simulink model "bh_4bar_model_KIN"  (R2019a)
settings: Solver=ode45  StartTime=0.0  StopTime=20  MaxStep=0.1  RelTol=1e-3  EnableMultiTasking=on
values from neighbouring files (symbols this model uses):
  L1 = 0.4    [bh_4bar_kin_z_analysis_CLS.m]
  L2 = 1.4    [bh_4bar_kin_z_analysis_CLS.m]
  L3 = 1.2    [bh_4bar_kin_z_analysis_CLS.m]
  L4 = 1    [bh_4bar_kin_z_analysis_CLS.m]
  N = length(THE_DEG_ANG_VEC)    [bh_4bar_kin_z_analysis_CLS.m]
  X = my_stuff_T.theta_deg_vec    [bh_4bar_kin_z_analysis_CLS.m]
undefined symbols (not defined in the file or in its folder): H, joints, theta_0_rad, W, Y, Z
libraries: nesl_utility x27, sm_lib x17, simulink_extras x7, bh_4bar_SL_LIB x7, simulink x1
settings Model: EnablePacing=on  Creator=bhorton  LastModifiedBy=bhorton
settings DataIOCC: LimitDataPoints=on  ReturnWorkspaceOutputs=off
settings OptimizationCC: LifeSpan=inf
settings DebuggingCC: AllowSymbolicDim=off  PregeneratedLibrarySubsystemCodeDiagnostic=none  SFUnexpectedBacktrackingDiag=warning  SFNoUnconditionalDefaultTransitionDiag=warning  SFExecutionAtInitializationDiag=none  ArithmeticOperatorsInVariantConditions=warning
settings SFSimCC: SimUseLocalCustomCode=off
settings RTWCC: RTWUseLocalCustomCode=off
settings CodeAppCC: StateflowObjectComments=on
settings GRTTargetCC: TargetLangStandard=C89/C90 (ANSI)  GeneratePreprocessorConditionals=Disable all
settings ConfigComp: CovMetricSettings=dw  CovHtmlReporting=on  CovSaveCumulativeToWorkspaceVar=on  CovSaveSingleToWorkspaceVar=on  CovExternalEMLEnable=off  CovSFcnEnable=off
settings SimscapeCC: SimscapeNominalValues="[{\"value\":\"10\",\"unit\":\"V\"},{\"value\":\"1\",\"unit\":\"A\"},{\"value\":\"10\",\"unit\":\"N*m\"},{\"value\":\"10\",\"unit\":\"bar\"},{\"value\":\"100\",\"unit\":\"kJ/kg\"},{\"value\":\"1\",\"unit\":\"kW\"},{\"value\":\"300\",\"unit\":\"K\"},{\"value\":\"100\",\"unit\":\"cm^3/s\"},{\"value\":\"1\",\"unit\":\"kN\"},{\"value\":\"1\",\"unit\":\"g/cm^3\"},{\"value\":\"1\",\"unit\":\"l\"},{\"value\":\"1\",\"unit\":\"cm^2\"},{\"value\":\"60\",\"unit\":\"Hz\"}]"  SimscapeLogType=all  SimscapeLogDataHistory=10000
settings ConfigurationSet: Description=SimMechanics 2G
settings ExplorerConfigSet: InternalSimMechanicsExplorerSettings="<ExplorerConfiguration><canonicalview>default</canonicalview><AnimationSetting><BasePlaybackSpeed>1.0</BasePlaybackSpeed><PlaybackSpeedFactor>1.0</PlaybackSpeedFactor></AnimationSetting><TilePanel><TileInfo><Tiles Columns=\"1\" Count=\"1\" Rows=\"1\"><Column Weight=\"1\"/><Row Weight=\"1\"/><Tile Height=\"1\" Width=\"1\" X=\"0\" Y=\"0\"/></Tiles></TileInfo><SceneInfo><SceneViewer><BGColor><R>0.60000002384185791</R><G>0.60000002384185791</G><B>0.60000002384185791</B></BGColor><Camera><DoPerspective>off</DoPerspective><Position><X>0.027900076379062555</X><Y>-0.43953442521543673</Y><Z>1.15928585903234671</Z></Position><Center><X>0.027900076379062555</X><Y>-0.43953442521543673</Y><Z>-0.00499998996240980098</Z></Center><Up><X>0</X><Y>1</Y><Z>-0</Z></Up><ViewLimDist>1</ViewLimDist><YLim>2.16648122412032906</YLim><XLim>2.57652145580412029</XLim></Camera></SceneViewer></SceneInfo></TilePanel><MechEditorPanel><Cameras/><GfxPanelCameraMap/><VideoCreator><PlaybackSpeedRatio>1.0</PlaybackSpeedRatio><FrameRate>30</FrameRate><VideoFormat>Motion JPEG AVI</VideoFormat><FrameSize>auto</FrameSize></VideoCreator></MechEditorPanel></ExplorerConfiguration>"

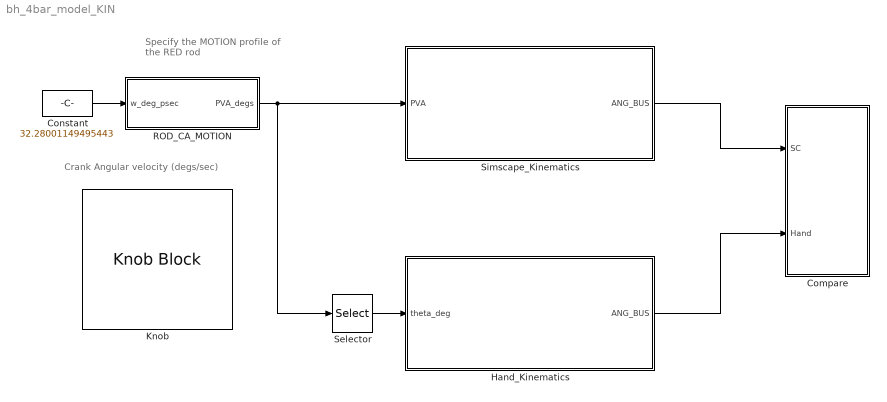
== system bh_4bar_model_KIN ==
  note: Crank Angular velocity (degs/sec)
  note: Specify the MOTION
      | profile of the RED rod
  Compare : Subsystem
  Constant : Constant  Value=32.28001149495443
  Hand_Kinematics : Subsystem
  Knob : KnobBlock
  ROD_CA_MOTION : Subsystem
  Selector : Selector  InputPortWidth=3  IndexOptions=Index vector (dialog)  Indices=1  OutputSizes=1
  Simscape_Kinematics : Subsystem
  wires:
  ROD_CA_MOTION/1(PVA_degs) -> Simscape_Kinematics/1(PVA), Selector/1
  Selector/1 -> Hand_Kinematics/1(theta_deg)
  Simscape_Kinematics/1(ANG_BUS) -> Compare/1(SC)
  Hand_Kinematics/1(ANG_BUS) -> Compare/2(Hand)
  Constant/1 -> ROD_CA_MOTION/1(w_deg_psec)

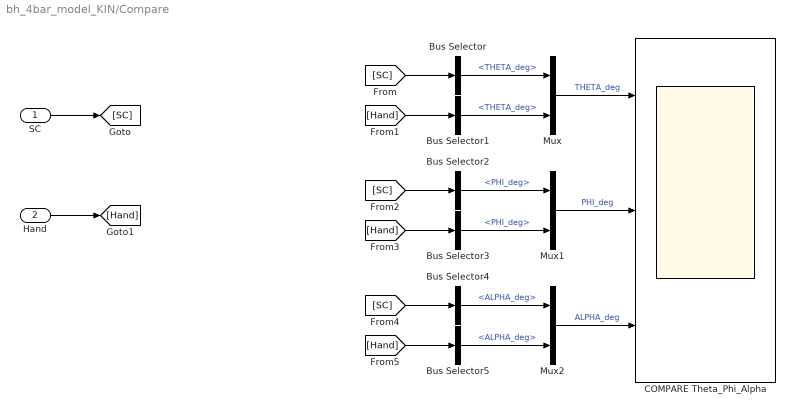
== system bh_4bar_model_KIN/Compare ==
  SC : Inport
  Hand : Inport  Port=2
  Bus Selector : BusSelector  OutputSignals=THETA_deg
  Bus Selector1 : BusSelector  OutputSignals=THETA_deg
  Bus Selector2 : BusSelector  OutputSignals=PHI_deg
  Bus Selector3 : BusSelector  OutputSignals=PHI_deg
  Bus Selector4 : BusSelector  OutputSignals=ALPHA_deg
  Bus Selector5 : BusSelector  OutputSignals=ALPHA_deg
  COMPARE Theta_Phi_Alpha : Scope  NumInputPorts=3
  Mux : Mux  Inputs=2
  Mux1 : Mux  Inputs=2
  Mux2 : Mux  Inputs=2
  wires:
  Hand/1 -> [Hand]
  SC/1 -> [SC]
  Mux/1 -> COMPARE Theta_Phi_Alpha/1  "THETA_deg"
  [SC] -> Bus Selector/1
  Bus Selector/1 -> Mux/1  "<THETA_deg>"
  [Hand] -> Bus Selector1/1
  Bus Selector1/1 -> Mux/2  "<THETA_deg>"
  Mux1/1 -> COMPARE Theta_Phi_Alpha/2  "PHI_deg"
  [SC] -> Bus Selector2/1
  Bus Selector3/1 -> Mux1/2  "<PHI_deg>"
  [Hand] -> Bus Selector3/1
  Bus Selector2/1 -> Mux1/1  "<PHI_deg>"
  Mux2/1 -> COMPARE Theta_Phi_Alpha/3  "ALPHA_deg"
  [Hand] -> Bus Selector5/1
  [SC] -> Bus Selector4/1
  Bus Selector5/1 -> Mux2/2  "<ALPHA_deg>"
  Bus Selector4/1 -> Mux2/1  "<ALPHA_deg>"

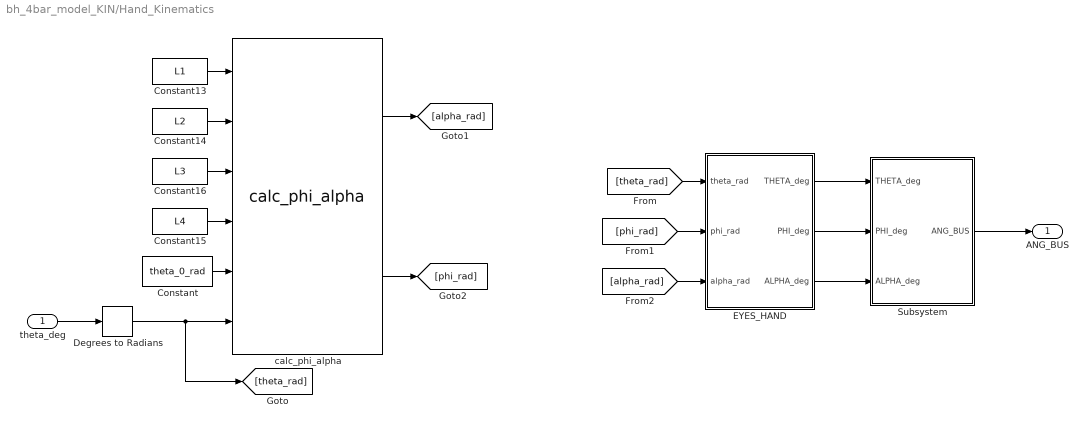
== system bh_4bar_model_KIN/Hand_Kinematics ==
  theta_deg : Inport
  Constant : Constant  Value=theta_0_rad
  Constant13 : Constant  Value=L1
  Constant14 : Constant  Value=L2
  Constant15 : Constant  Value=L4
  Constant16 : Constant  Value=L3
  Degrees to Radians : simulink_extras/Transformations/Degrees to Radians
  EYES_HAND : Subsystem
  Subsystem : Subsystem
  calc_phi_alpha : bh_4bar_SL_LIB/4bar_basics/calc_phi_alpha  SystemSampleTime=-1
  ANG_BUS : Outport
  wires:
  Constant14/1 -> calc_phi_alpha/2
  Constant13/1 -> calc_phi_alpha/1
  Constant15/1 -> calc_phi_alpha/4
  Constant16/1 -> calc_phi_alpha/3
  Degrees to Radians/1 -> [theta_rad], calc_phi_alpha/6
  theta_deg/1 -> Degrees to Radians/1
  EYES_HAND/1(THETA_deg) -> Subsystem/1(THETA_deg)
  EYES_HAND/3(ALPHA_deg) -> Subsystem/3(ALPHA_deg)
  EYES_HAND/2(PHI_deg) -> Subsystem/2(PHI_deg)
  [phi_rad] -> EYES_HAND/2(phi_rad)
  Subsystem/1(ANG_BUS) -> ANG_BUS/1
  [alpha_rad] -> EYES_HAND/3(alpha_rad)
  [theta_rad] -> EYES_HAND/1(theta_rad)
  calc_phi_alpha/2 -> [phi_rad]
  calc_phi_alpha/1 -> [alpha_rad]
  Constant/1 -> calc_phi_alpha/5

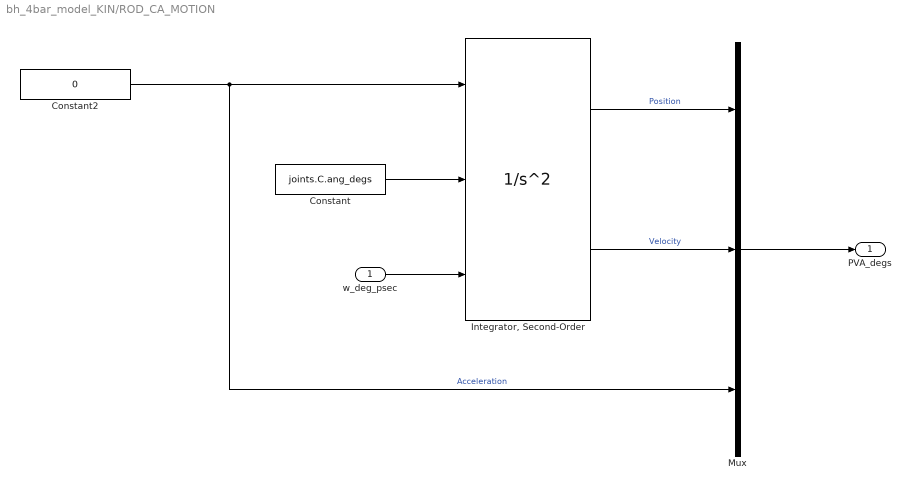
== system bh_4bar_model_KIN/ROD_CA_MOTION ==
  w_deg_psec : Inport
  Constant : Constant  Value=joints.C.ang_degs
  Constant2 : Constant  Value=0
  "Integrator, Second-Order" : SecondOrderIntegrator  ICSourceX=external  ICSourceDXDT=external
  Mux : Mux  Inputs=3
  PVA_degs : Outport
  wires:
  Constant2/1 -> Mux/3, "Integrator, Second-Order"/1  "Acceleration"
  w_deg_psec/1 -> "Integrator, Second-Order"/3
  Constant/1 -> "Integrator, Second-Order"/2
  "Integrator, Second-Order"/1 -> Mux/1  "Position"
  "Integrator, Second-Order"/2 -> Mux/2  "Velocity"
  Mux/1 -> PVA_degs/1

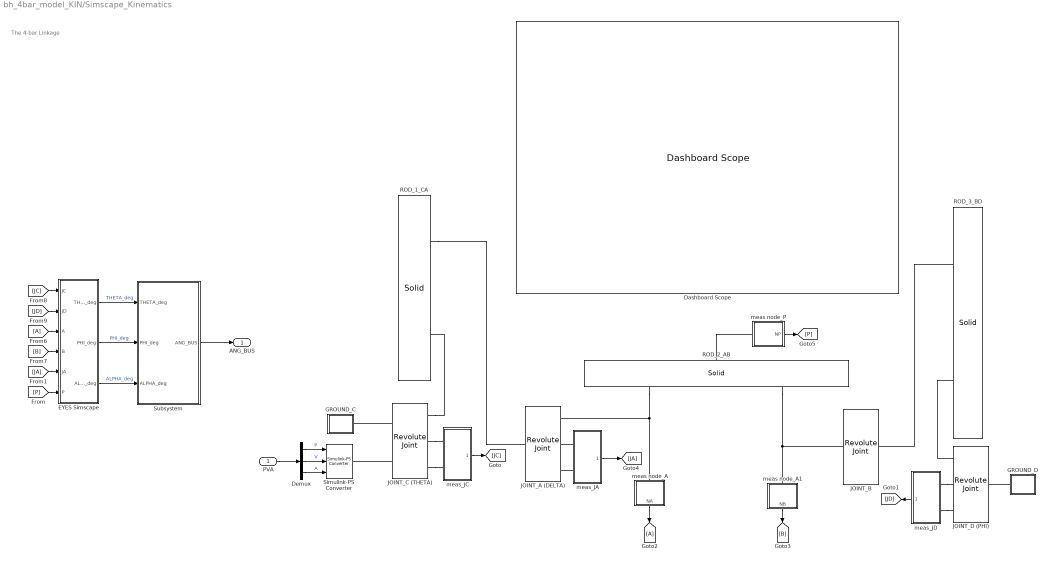
== system bh_4bar_model_KIN/Simscape_Kinematics ==
  note: The 4-bar Linkage
  PVA : Inport
  Dashboard Scope : DashboardScope
  Demux : Demux  Outputs=3
  EYES Simscape : Subsystem
  GROUND_C : Subsystem
  GROUND_D : Subsystem
  JOINT_A (DELTA) : sm_lib/Joints/Revolute Joint  SenseConstraintForce=off  SenseConstraintForceX=off  SenseConstraintForceY=off  SenseConstraintForceZ=off  SenseConstraintTorque=off  SenseConstraintTorqueX=off  SenseConstraintTorqueY=off  SenseConstraintTorqueZ=off  SenseTotalForce=off  SenseTotalForceX=off  SenseTotalForceY=off  SenseTotalForceZ=off  SenseTotalTorque=off  SenseTotalTorqueX=off  SenseTotalTorqueY=off  SenseTotalTorqueZ=off  CompositeWrenchDir=FollowerOnBase  CompositeWrenchFrame=BaseFrame  EquilibriumPosition=0  EquilibriumPositionUnits=deg  SpringStiffness=0  SpringStiffnessUnits=N*m/deg  DampingCoefficient=0  DampingCoefficientUnits=N*m/(deg/s)  TorqueActuationMode=NoTorque  MotionActuationMode=ComputedMotion  SensePosition=on  SenseVelocity=on  SenseAcceleration=off  SenseTorqueForce=off  SenseLowerLimitTorqueForce=off  SenseUpperLimitTorqueForce=off  LowerLimitSpecify=off  LowerLimitBound=-90  LowerLimitBoundUnits=deg  LowerLimitStiffness=1e4  LowerLimitStiffnessUnits=N*m/deg  LowerLimitDamping=10  LowerLimitDampingUnits=N*m/(deg/s)  LowerLimitTransitionRegionWidth=0.1  LowerLimitTransitionRegionWidthUnits=deg  UpperLimitSpecify=off  UpperLimitBound=90  UpperLimitBoundUnits=deg  UpperLimitStiffness=1e4  UpperLimitStiffnessUnits=N*m/deg  UpperLimitDamping=10  UpperLimitDampingUnits=N*m/(deg/s)  UpperLimitTransitionRegionWidth=0.1  UpperLimitTransitionRegionWidthUnits=deg  PositionTargetSpecify=off  PositionTargetPriority=High  PositionTargetValue=0  PositionTargetValueUnits=deg  VelocityTargetSpecify=off  VelocityTargetPriority=High  VelocityTargetValue=0  VelocityTargetValueUnits=deg/s
  JOINT_B : sm_lib/Joints/Revolute Joint  SenseConstraintForce=off  SenseConstraintForceX=off  SenseConstraintForceY=off  SenseConstraintForceZ=off  SenseConstraintTorque=off  SenseConstraintTorqueX=off  SenseConstraintTorqueY=off  SenseConstraintTorqueZ=off  SenseTotalForce=off  SenseTotalForceX=off  SenseTotalForceY=off  SenseTotalForceZ=off  SenseTotalTorque=off  SenseTotalTorqueX=off  SenseTotalTorqueY=off  SenseTotalTorqueZ=off  CompositeWrenchDir=FollowerOnBase  CompositeWrenchFrame=BaseFrame  EquilibriumPosition=0  EquilibriumPositionUnits=deg  SpringStiffness=0  SpringStiffnessUnits=N*m/deg  DampingCoefficient=0  DampingCoefficientUnits=N*m/(deg/s)  TorqueActuationMode=NoTorque  MotionActuationMode=ComputedMotion  SensePosition=off  SenseVelocity=off  SenseAcceleration=off  SenseTorqueForce=off  SenseLowerLimitTorqueForce=off  SenseUpperLimitTorqueForce=off  LowerLimitSpecify=off  LowerLimitBound=-90  LowerLimitBoundUnits=deg  LowerLimitStiffness=1e4  LowerLimitStiffnessUnits=N*m/deg  LowerLimitDamping=10  LowerLimitDampingUnits=N*m/(deg/s)  LowerLimitTransitionRegionWidth=0.1  LowerLimitTransitionRegionWidthUnits=deg  UpperLimitSpecify=off  UpperLimitBound=90  UpperLimitBoundUnits=deg  UpperLimitStiffness=1e4  UpperLimitStiffnessUnits=N*m/deg  UpperLimitDamping=10  UpperLimitDampingUnits=N*m/(deg/s)  UpperLimitTransitionRegionWidth=0.1  UpperLimitTransitionRegionWidthUnits=deg  PositionTargetSpecify=off  PositionTargetPriority=High  PositionTargetValue=0  PositionTargetValueUnits=deg  VelocityTargetSpecify=off  VelocityTargetPriority=High  VelocityTargetValue=0  VelocityTargetValueUnits=deg/s
  JOINT_C (THETA) : sm_lib/Joints/Revolute Joint  SenseConstraintForce=off  SenseConstraintForceX=off  SenseConstraintForceY=off  SenseConstraintForceZ=off  SenseConstraintTorque=off  SenseConstraintTorqueX=off  SenseConstraintTorqueY=off  SenseConstraintTorqueZ=off  SenseTotalForce=off  SenseTotalForceX=off  SenseTotalForceY=off  SenseTotalForceZ=off  SenseTotalTorque=off  SenseTotalTorqueX=off  SenseTotalTorqueY=off  SenseTotalTorqueZ=off  CompositeWrenchDir=FollowerOnBase  CompositeWrenchFrame=BaseFrame  EquilibriumPosition=0  EquilibriumPositionUnits=deg  SpringStiffness=0  SpringStiffnessUnits=N*m/deg  DampingCoefficient=0  DampingCoefficientUnits=N*m/(deg/s)  TorqueActuationMode=ComputedTorque  MotionActuationMode=InputMotion  SensePosition=on  SenseVelocity=on  SenseAcceleration=off  SenseTorqueForce=off  SenseLowerLimitTorqueForce=off  SenseUpperLimitTorqueForce=off  LowerLimitSpecify=off  LowerLimitBound=-90  LowerLimitBoundUnits=deg  LowerLimitStiffness=1e4  LowerLimitStiffnessUnits=N*m/deg  LowerLimitDamping=10  LowerLimitDampingUnits=N*m/(deg/s)  LowerLimitTransitionRegionWidth=0.1  LowerLimitTransitionRegionWidthUnits=deg  UpperLimitSpecify=off  UpperLimitBound=90  UpperLimitBoundUnits=deg  UpperLimitStiffness=1e4  UpperLimitStiffnessUnits=N*m/deg  UpperLimitDamping=10  UpperLimitDampingUnits=N*m/(deg/s)  UpperLimitTransitionRegionWidth=0.1  UpperLimitTransitionRegionWidthUnits=deg  PositionTargetSpecify=on  PositionTargetPriority=High  PositionTargetValue=joints.C.ang_degs  PositionTargetValueUnits=deg  VelocityTargetSpecify=on  VelocityTargetPriority=High  VelocityTargetValue=joints.C.vel_degs  VelocityTargetValueUnits=deg/s
      settings: AttributesFormatString=|
      | init_pos =%<PositionTargetValue>
      | %<PositionTargetValueUnits>
  JOINT_D (PHI) : sm_lib/Joints/Revolute Joint  SenseConstraintForce=off  SenseConstraintForceX=off  SenseConstraintForceY=off  SenseConstraintForceZ=off  SenseConstraintTorque=off  SenseConstraintTorqueX=off  SenseConstraintTorqueY=off  SenseConstraintTorqueZ=off  SenseTotalForce=off  SenseTotalForceX=off  SenseTotalForceY=off  SenseTotalForceZ=off  SenseTotalTorque=off  SenseTotalTorqueX=off  SenseTotalTorqueY=off  SenseTotalTorqueZ=off  CompositeWrenchDir=FollowerOnBase  CompositeWrenchFrame=BaseFrame  EquilibriumPosition=0  EquilibriumPositionUnits=deg  SpringStiffness=0  SpringStiffnessUnits=N*m/deg  DampingCoefficient=0  DampingCoefficientUnits=N*m/(deg/s)  TorqueActuationMode=NoTorque  MotionActuationMode=ComputedMotion  SensePosition=on  SenseVelocity=on  SenseAcceleration=off  SenseTorqueForce=off  SenseLowerLimitTorqueForce=off  SenseUpperLimitTorqueForce=off  LowerLimitSpecify=off  LowerLimitBound=-90  LowerLimitBoundUnits=deg  LowerLimitStiffness=1e4  LowerLimitStiffnessUnits=N*m/deg  LowerLimitDamping=10  LowerLimitDampingUnits=N*m/(deg/s)  LowerLimitTransitionRegionWidth=0.1  LowerLimitTransitionRegionWidthUnits=deg  UpperLimitSpecify=off  UpperLimitBound=90  UpperLimitBoundUnits=deg  UpperLimitStiffness=1e4  UpperLimitStiffnessUnits=N*m/deg  UpperLimitDamping=10  UpperLimitDampingUnits=N*m/(deg/s)  UpperLimitTransitionRegionWidth=0.1  UpperLimitTransitionRegionWidthUnits=deg  PositionTargetSpecify=on  PositionTargetPriority=High  PositionTargetValue=joints.D.ang_degs  PositionTargetValueUnits=deg  VelocityTargetSpecify=off  VelocityTargetPriority=High  VelocityTargetValue=0  VelocityTargetValueUnits=deg/s
      settings: AttributesFormatString=|
      | init_pos =%<PositionTargetValue>
      | %<PositionTargetValueUnits>
  ROD_1_CA : sm_lib/Body Elements/Solid  InertiaType=CalculateFromGeometry  Mass=1  MassUnits=kg  CenterOfMass=[0 0 0]  CenterOfMassUnits=m  MomentsOfInertia=[1 1 1]  MomentsOfInertiaUnits=kg*m^2  ProductsOfInertia=[0 0 0]  ProductsOfInertiaUnits=kg*m^2  BasedOnType=Density  Density=density  DensityUnits=kg/m^3  DoExposeReferenceFrame=on  SerializedFrames=<Frames><Frame><Id>Frame2</Id><Value><Name>A</Name><Origin><Source>GeometricFeature</Source><FeatureName>+z +x curve</FeatureName></Origin><PrimaryAxis><DefinedDirection>+Z</DefinedDirection><Source>ReferenceFrame</Source><SourceDirection>+Z</SourceDirection><FeatureName></FeatureName></PrimaryAxis><SecondaryAxis><DefinedDirection>+X</DefinedDirection><Source>ReferenceFrame</Source><SourceDirection>+X</SourceDirection><FeatureName></FeatureName></SecondaryAxis></Value></Frame><Frame><Id>Frame3</Id><Value><Name>C</Name><Origin><Source>GeometricFeature</Source><FeatureName>+z -x curve</FeatureName></Origin><PrimaryAxis><DefinedDirection>+Z</DefinedDirection><Source>ReferenceFrame</Source><SourceDirection>+Z</SourceDirection><FeatureName></FeatureName></PrimaryAxis><SecondaryAxis><DefinedDirection>+X</DefinedDirection><Source>ReferenceFrame</Source><SourceDirection>+X</SourceDirection><FeatureName></FeatureName></SecondaryAxis></Value></Frame></Frames>  GraphicType=FromGeometry  MarkerShape=Sphere  MarkerSize=10  GraphicVisPropType=SimpleVisualProperties  GraphicDiffuseColor=[1.0 0.4 0.6]  GraphicSpecularColor=[0.5 0.5 0.5 1.0]  GraphicAmbientColor=[0.15 0.15 0.15 1.0]  GraphicEmissiveColor=[0.0 0.0 0.0 1.0]  GraphicShininess=75  GraphicOpacity=1.0  GeometryShape=Brick  RectangleSize=[1 1]  RectangleSizeUnits=m  BrickDimensions=[L1,H,W]  BrickDimensionUnits=m  CylinderRadius=1  CylinderRadiusUnits=m  CylinderLength=1  CylinderLengthUnits=m  SphereRadius=1  SphereRadiusUnits=m  EllipsoidRadii=[1 1 1]  EllipsoidRadiiUnits=m  ExtrusionCrossSection=[1 1; -1 1; -1 -1; 1 -1]  ExtrusionCrossSectionUnits=m  ExtrusionLength=1  ExtrusionLengthUnits=m  PolygonNumSides=3  PolygonOuterRadius=1  PolygonOuterRadiusUnits=m  ExtGeomFileType=STEP  ExtGeomFileUnits=m  RevolutionCrossSection=[1 1; 1 -1; 2 -1; 2 1]  RevolutionCrossSectionUnits=m  RevolutionExtent=Full  RevolutionAngle=180  RevolutionAngleUnits=deg
  ROD_2_AB : sm_lib/Body Elements/Solid  InertiaType=CalculateFromGeometry  Mass=1  MassUnits=kg  CenterOfMass=[0 0 0]  CenterOfMassUnits=m  MomentsOfInertia=[1 1 1]  MomentsOfInertiaUnits=kg*m^2  ProductsOfInertia=[0 0 0]  ProductsOfInertiaUnits=kg*m^2  BasedOnType=Density  Density=density  DensityUnits=kg/m^3  DoExposeReferenceFrame=on  SerializedFrames=<Frames><Frame><Id>Frame1</Id><Value><Name>A</Name><Origin><Source>GeometricFeature</Source><FeatureName>+z -x curve</FeatureName></Origin><PrimaryAxis><DefinedDirection>+Z</DefinedDirection><Source>ReferenceFrame</Source><SourceDirection>+Z</SourceDirection><FeatureName></FeatureName></PrimaryAxis><SecondaryAxis><DefinedDirection>+X</DefinedDirection><Source>ReferenceFrame</Source><SourceDirection>+X</SourceDirection><FeatureName></FeatureName></SecondaryAxis></Value></Frame><Frame><Id>Frame2</Id><Value><Name>B</Name><Origin><Source>GeometricFeature</Source><FeatureName>+z +x curve</FeatureName></Origin><PrimaryAxis><DefinedDirection>+Z</DefinedDirection><Source>ReferenceFrame</Source><SourceDirection>+Z</SourceDirection><FeatureName></FeatureName></PrimaryAxis><SecondaryAxis><DefinedDirection>+X</DefinedDirection><Source>ReferenceFrame</Source><SourceDirection>+X</SourceDirection><FeatureName></FeatureName></SecondaryAxis></Value></Frame></Frames>  GraphicType=FromGeometry  MarkerShape=Sphere  MarkerSize=10  GraphicVisPropType=SimpleVisualProperties  GraphicDiffuseColor=[0.0 1.0 0.2]  GraphicSpecularColor=[0.5 0.5 0.5 1.0]  GraphicAmbientColor=[0.15 0.15 0.15 1.0]  GraphicEmissiveColor=[0.0 0.0 0.0 1.0]  GraphicShininess=75  GraphicOpacity=1.0  GeometryShape=Brick  RectangleSize=[1 1]  RectangleSizeUnits=m  BrickDimensions=[L2,H,W]  BrickDimensionUnits=m  CylinderRadius=1  CylinderRadiusUnits=m  CylinderLength=1  CylinderLengthUnits=m  SphereRadius=1  SphereRadiusUnits=m  EllipsoidRadii=[1 1 1]  EllipsoidRadiiUnits=m  ExtrusionCrossSection=[1 1; -1 1; -1 -1; 1 -1]  ExtrusionCrossSectionUnits=m  ExtrusionLength=1  ExtrusionLengthUnits=m  PolygonNumSides=3  PolygonOuterRadius=1  PolygonOuterRadiusUnits=m  ExtGeomFileType=STEP  ExtGeomFileUnits=m  RevolutionCrossSection=[1 1; 1 -1; 2 -1; 2 1]  RevolutionCrossSectionUnits=m  RevolutionExtent=Full  RevolutionAngle=180  RevolutionAngleUnits=deg
  ROD_3_BD : sm_lib/Body Elements/Solid  InertiaType=CalculateFromGeometry  Mass=1  MassUnits=kg  CenterOfMass=[0 0 0]  CenterOfMassUnits=m  MomentsOfInertia=[1 1 1]  MomentsOfInertiaUnits=kg*m^2  ProductsOfInertia=[0 0 0]  ProductsOfInertiaUnits=kg*m^2  BasedOnType=Density  Density=density  DensityUnits=kg/m^3  DoExposeReferenceFrame=on  SerializedFrames=<Frames><Frame><Id>Frame1</Id><Value><Name>B</Name><Origin><Source>GeometricFeature</Source><FeatureName>+z +x curve</FeatureName></Origin><PrimaryAxis><DefinedDirection>+Z</DefinedDirection><Source>ReferenceFrame</Source><SourceDirection>+Z</SourceDirection><FeatureName></FeatureName></PrimaryAxis><SecondaryAxis><DefinedDirection>+X</DefinedDirection><Source>ReferenceFrame</Source><SourceDirection>+X</SourceDirection><FeatureName></FeatureName></SecondaryAxis></Value></Frame><Frame><Id>Frame2</Id><Value><Name>D</Name><Origin><Source>GeometricFeature</Source><FeatureName>+z -x curve</FeatureName></Origin><PrimaryAxis><DefinedDirection>+Z</DefinedDirection><Source>ReferenceFrame</Source><SourceDirection>+Z</SourceDirection><FeatureName></FeatureName></PrimaryAxis><SecondaryAxis><DefinedDirection>+X</DefinedDirection><Source>ReferenceFrame</Source><SourceDirection>+X</SourceDirection><FeatureName></FeatureName></SecondaryAxis></Value></Frame></Frames>  GraphicType=FromGeometry  MarkerShape=Sphere  MarkerSize=10  GraphicVisPropType=SimpleVisualProperties  GraphicDiffuseColor=[0.2 0.2 1.0]  GraphicSpecularColor=[0.5 0.5 0.5 1.0]  GraphicAmbientColor=[0.15 0.15 0.15 1.0]  GraphicEmissiveColor=[0.0 0.0 0.0 1.0]  GraphicShininess=75  GraphicOpacity=1.0  GeometryShape=Brick  RectangleSize=[1 1]  RectangleSizeUnits=m  BrickDimensions=[L3,H,W]  BrickDimensionUnits=m  CylinderRadius=1  CylinderRadiusUnits=m  CylinderLength=1  CylinderLengthUnits=m  SphereRadius=1  SphereRadiusUnits=m  EllipsoidRadii=[1 1 1]  EllipsoidRadiiUnits=m  ExtrusionCrossSection=[1 1; -1 1; -1 -1; 1 -1]  ExtrusionCrossSectionUnits=m  ExtrusionLength=1  ExtrusionLengthUnits=m  PolygonNumSides=3  PolygonOuterRadius=1  PolygonOuterRadiusUnits=m  ExtGeomFileType=STEP  ExtGeomFileUnits=m  RevolutionCrossSection=[1 1; 1 -1; 2 -1; 2 1]  RevolutionCrossSectionUnits=m  RevolutionExtent=Full  RevolutionAngle=180  RevolutionAngleUnits=deg
  Simulink-PS Converter : nesl_utility/Simulink-PS Converter  PhysicalDomain=network_engine_domain  SubClassName=ps_input  LeftPortType=input  RightPortType=output  PseudoPeriodic=off  Frequencies=[]  NoiseDistribution=none  NoiseParameters=[]  Unit=deg  AffineConversion=off  FilteringAndDerivatives=provide  SimscapeFilterOrder=1  InputFilterTimeConstant=0.001  UdotUserProvided=2
  Subsystem : Subsystem
  meas node_A : Subsystem
  meas node_A1 : Subsystem
  meas node_P : Subsystem
  meas_JA : Subsystem
  meas_JC : Subsystem
  meas_JD : Subsystem
  ANG_BUS : Outport
  wires:
  EYES Simscape/1(THETA_deg) -> Subsystem/1(THETA_deg)  "THETA_deg"
  Demux/2 -> Simulink-PS Converter/2  "V"
  Demux/1 -> Simulink-PS Converter/1  "P"
  meas_JD/1(PV_BUS) -> [JD]
  meas node_A/1(NA) -> [A]
  Subsystem/1(ANG_BUS) -> ANG_BUS/1
  [A] -> EYES Simscape/3(A)
  meas node_A1/1(NB) -> [B]
  [JA] -> EYES Simscape/5(JA)
  PVA/1 -> Demux/1
  meas_JC/1(PV_BUS) -> [JC]
  [JD] -> EYES Simscape/2(JD)
  Demux/3 -> Simulink-PS Converter/3  "A"
  EYES Simscape/2(PHI_deg) -> Subsystem/2(PHI_deg)  "PHI_deg"
  meas_JA/1(PV_BUS) -> [JA]
  [JC] -> EYES Simscape/1(JC)
  [B] -> EYES Simscape/4(B)
  EYES Simscape/3(ALPHA_deg) -> Subsystem/3(ALPHA_deg)  "ALPHA_deg"
  meas node_P/1(NP) -> [P]
  [P] -> EYES Simscape/6(P)
  connections:
  meas node_A/LConn1 -- ROD_2_AB/LConn1 -- JOINT_A (DELTA)/RConn1
  ROD_3_BD/LConn1 -- JOINT_B/RConn1
  JOINT_C (THETA)/LConn2 -- Simulink-PS Converter/RConn1
  JOINT_D (PHI)/RConn1 -- ROD_3_BD/LConn2
  ROD_2_AB/LConn2 -- meas node_A1/LConn1 -- JOINT_B/LConn1
  GROUND_D/RConn1 -- JOINT_D (PHI)/LConn1
  JOINT_C (THETA)/LConn1 -- GROUND_C/RConn1
  meas_JA/LConn1 -- JOINT_A (DELTA)/RConn2
  JOINT_C (THETA)/RConn3 -- meas_JC/LConn2
  meas_JD/LConn2 -- JOINT_D (PHI)/RConn3
  JOINT_C (THETA)/RConn2 -- meas_JC/LConn1
  meas_JD/LConn1 -- JOINT_D (PHI)/RConn2
  meas_JA/LConn2 -- JOINT_A (DELTA)/RConn3
  ROD_1_CA/LConn1 -- JOINT_A (DELTA)/LConn1
  JOINT_C (THETA)/RConn1 -- ROD_1_CA/LConn2
  ROD_2_AB/RConn1 -- meas node_P/LConn1

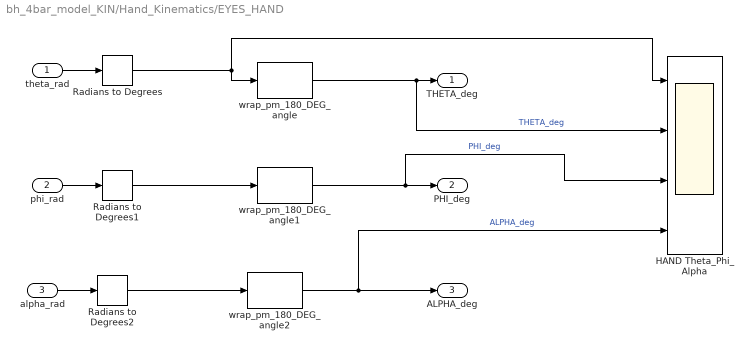
== system bh_4bar_model_KIN/Hand_Kinematics/EYES_HAND ==
  theta_rad : Inport
  phi_rad : Inport  Port=2
  alpha_rad : Inport  Port=3
  HAND Theta_Phi_Alpha : Scope  NumInputPorts=4
  Radians to Degrees : simulink_extras/Transformations/Radians to Degrees
  Radians to Degrees1 : simulink_extras/Transformations/Radians to Degrees
  Radians to Degrees2 : simulink_extras/Transformations/Radians to Degrees
  wrap_pm_180_DEG_angle : bh_4bar_SL_LIB/4bar_basics/wrap_pm_180_DEG_angle  SystemSampleTime=-1
  wrap_pm_180_DEG_angle1 : bh_4bar_SL_LIB/4bar_basics/wrap_pm_180_DEG_angle  SystemSampleTime=-1
  wrap_pm_180_DEG_angle2 : bh_4bar_SL_LIB/4bar_basics/wrap_pm_180_DEG_angle  SystemSampleTime=-1
  THETA_deg : Outport
  PHI_deg : Outport  Port=2
  ALPHA_deg : Outport  Port=3
  wires:
  theta_rad/1 -> Radians to Degrees/1
  alpha_rad/1 -> Radians to Degrees2/1
  phi_rad/1 -> Radians to Degrees1/1
  Radians to Degrees/1 -> wrap_pm_180_DEG_angle/1, HAND Theta_Phi_Alpha/1
  Radians to Degrees1/1 -> wrap_pm_180_DEG_angle1/1
  Radians to Degrees2/1 -> wrap_pm_180_DEG_angle2/1
  wrap_pm_180_DEG_angle/1 -> HAND Theta_Phi_Alpha/2, THETA_deg/1  "THETA_deg"
  wrap_pm_180_DEG_angle1/1 -> HAND Theta_Phi_Alpha/3, PHI_deg/1  "PHI_deg"
  wrap_pm_180_DEG_angle2/1 -> HAND Theta_Phi_Alpha/4, ALPHA_deg/1  "ALPHA_deg"

== system bh_4bar_model_KIN/Hand_Kinematics/Subsystem ==
  THETA_deg : Inport
  PHI_deg : Inport  Port=2
  ALPHA_deg : Inport  Port=3
  Bus Creator : BusCreator  Inputs=3
  ANG_BUS : Outport
  wires:
  ALPHA_deg/1 -> Bus Creator/3  "ALPHA_deg"
  PHI_deg/1 -> Bus Creator/2  "PHI_deg"
  THETA_deg/1 -> Bus Creator/1  "THETA_deg"
  Bus Creator/1 -> ANG_BUS/1

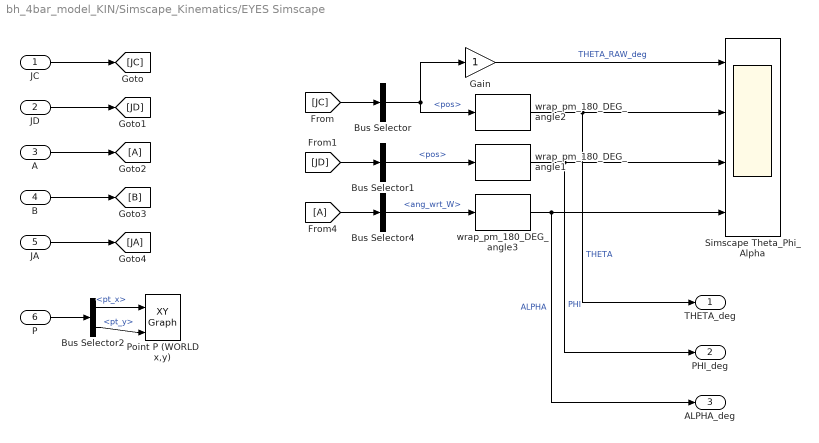
== system bh_4bar_model_KIN/Simscape_Kinematics/EYES Simscape ==
  JC : Inport
  JD : Inport  Port=2
  A : Inport  Port=3
  B : Inport  Port=4
  JA : Inport  Port=5
  P : Inport  Port=6
  Bus Selector : BusSelector  OutputSignals=pos
  Bus Selector1 : BusSelector  OutputSignals=pos
  Bus Selector2 : BusSelector  OutputSignals=pt_x,pt_y
  Bus Selector4 : BusSelector  OutputSignals=ang_wrt_W
  Gain : Gain
  Point P (WORLD x,y) : simulink/Sinks/XY Graph  xmin=-1*(L1+0.5*L2)  xmax=(L1+0.5*L2)  ymin=-1*max([L1, L3])  ymax=max([L1, L3])  st=-1
  Simscape Theta_Phi_Alpha : Scope  NumInputPorts=4
  wrap_pm_180_DEG_angle1 : bh_4bar_SL_LIB/4bar_basics/wrap_pm_180_DEG_angle  SystemSampleTime=-1
  wrap_pm_180_DEG_angle2 : bh_4bar_SL_LIB/4bar_basics/wrap_pm_180_DEG_angle  SystemSampleTime=-1
  wrap_pm_180_DEG_angle3 : bh_4bar_SL_LIB/4bar_basics/wrap_pm_180_DEG_angle  SystemSampleTime=-1
  THETA_deg : Outport
  PHI_deg : Outport  Port=2
  ALPHA_deg : Outport  Port=3
  wires:
  B/1 -> [B]
  A/1 -> [A]
  JD/1 -> [JD]
  JC/1 -> [JC]
  [JD] -> Bus Selector1/1
  [JC] -> Bus Selector/1
  Bus Selector/1 -> wrap_pm_180_DEG_angle2/1, Gain/1  "<pos>"
  [A] -> Bus Selector4/1
  wrap_pm_180_DEG_angle2/1 -> THETA_deg/1, Simscape Theta_Phi_Alpha/2  "THETA"
  wrap_pm_180_DEG_angle1/1 -> PHI_deg/1, Simscape Theta_Phi_Alpha/3  "PHI"
  JA/1 -> [JA]
  wrap_pm_180_DEG_angle3/1 -> ALPHA_deg/1, Simscape Theta_Phi_Alpha/4  "ALPHA"
  Gain/1 -> Simscape Theta_Phi_Alpha/1  "THETA_RAW_deg"
  Bus Selector1/1 -> wrap_pm_180_DEG_angle1/1  "<pos>"
  Bus Selector4/1 -> wrap_pm_180_DEG_angle3/1  "<ang_wrt_W>"
  P/1 -> Bus Selector2/1
  Bus Selector2/1 -> Point P (WORLD x,y)/1  "<pt_x>"
  Bus Selector2/2 -> Point P (WORLD x,y)/2  "<pt_y>"

== system bh_4bar_model_KIN/Simscape_Kinematics/GROUND_C ==
  Mechanism Configuration : sm_lib/Utilities/Mechanism Configuration  UniformGravity=Constant  GravityVector=[0 0 0]  GravityUnits=m/s^2  LinearizationDelta=0.001
  Solver Configuration : nesl_utility/Solver Configuration  PhysicalDomain=network_engine_domain  SubClassName=solver  LeftPortType=input  RightPortType=generic  Tones=[]  Harmonics=[]  SimulateNoise=off  Profile=off  UseLocalSampling=off  EnableSwitchedLinearOptims=on  FrequencyDomain=off  UseCCode=off  RelTol=0.001  AbsTol=1e-06  MinStep=1e-09  ToWorkspace=off  RevertToSquareIcSolve=off  NumHomotopyIterations=100  PhasorMode=off  PhasorModeNumHarmonics=1  DoDC=off  ResidualTolerance=1e-09  UseLocalSolver=off  LocalSolverChoice=NE_BACKWARD_EULER_ADVANCER  LocalSolverSampleTime=0.001  DoFixedCost=off  MaxNonlinIter=3  MaxModeIter=2  LinearAlgebra=Sparse  EquationFormulation=NE_TIME_EF  DelaysMemoryBudget=1024  AutomaticFiltering=on  FilteringTimeConstant=0.001  PartitionStorageMethod=AS_NEEDED  PartitionMemoryBudget=1024  PartitionMethod=FAST
  World Frame : sm_lib/Frames and Transforms/World Frame
  Conn1 : PMIOPort  Side=Right
  connections:
  Solver Configuration/RConn1 -- Conn1/RConn1 -- Mechanism Configuration/RConn1 -- World Frame/RConn1

== system bh_4bar_model_KIN/Simscape_Kinematics/GROUND_D ==
  Rigid Transform : sm_lib/Frames and Transforms/Rigid Transform  TranslationMethod=StandardAxis  TranslationStandardOffset=L4  TranslationLengthUnit=m  TranslationStandardAxis=+X  TranslationCartesianOffset=[0 0 0]  TranslationROffset=0  TranslationROffsetUnits=m  TranslationZOffset=0  TranslationZOffsetUnits=m  TranslationThetaOffset=0  TranslationThetaOffsetUnits=deg  RotationMethod=None  RotationAngleUnits=deg  RotationStandardAxis=+Z  RotationAngle=0.0  RotationArbitraryAxis=[0 0 1]  FollAlignAxisA=+X  BaseAlignAxisA=+Y  FollAlignAxisB=+Y  BaseAlignAxisB=+Z  RotationSequenceAxes=FollowerAxes  RotationSequence=XYX  RotationSequenceAngles=[0 0 0]  RotationSequenceAnglesUnits=deg  RotationMatrix=[1 0 0; 0 1 0; 0 0 1]
  World Frame1 : sm_lib/Frames and Transforms/World Frame
  Conn1 : PMIOPort  Side=Right
  connections:
  Rigid Transform/LConn1 -- World Frame1/RConn1
  Rigid Transform/RConn1 -- Conn1/RConn1

== system bh_4bar_model_KIN/Simscape_Kinematics/Subsystem ==
  THETA_deg : Inport
  PHI_deg : Inport  Port=2
  ALPHA_deg : Inport  Port=3
  Bus Creator : BusCreator  Inputs=3
  ANG_BUS : Outport
  wires:
  ALPHA_deg/1 -> Bus Creator/3  "ALPHA_deg"
  PHI_deg/1 -> Bus Creator/2  "PHI_deg"
  THETA_deg/1 -> Bus Creator/1  "THETA_deg"
  Bus Creator/1 -> ANG_BUS/1

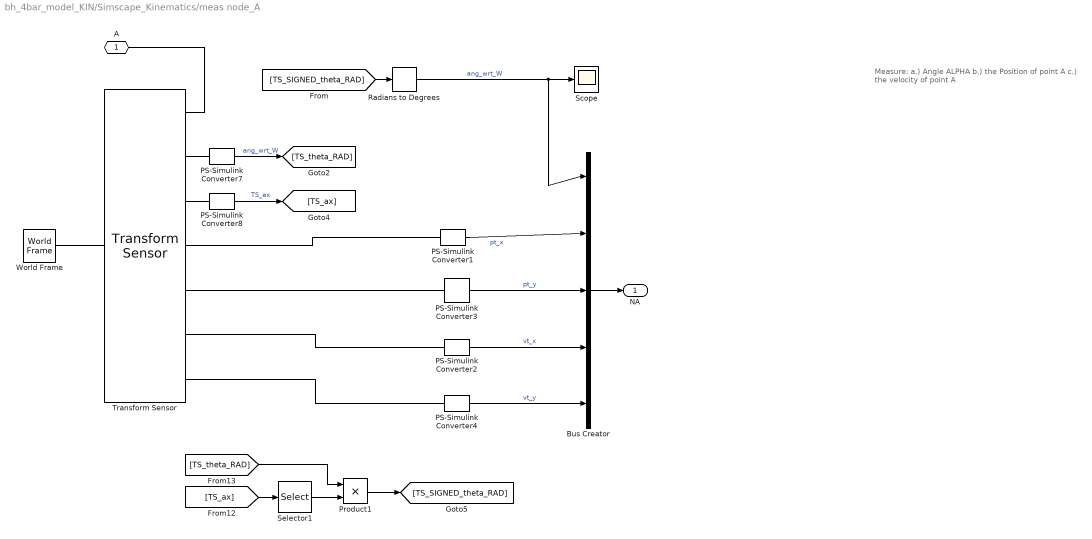
== system bh_4bar_model_KIN/Simscape_Kinematics/meas node_A ==
  note: Measure:
      | a.) Angle ALPHA
      | b.) the Position of point A
      | c.) the velocity of point A
  Bus Creator : BusCreator  Inputs=5
  PS-Simulink Converter1 : nesl_utility/PS-Simulink Converter  PhysicalDomain=network_engine_domain  SubClassName=ps_output  LeftPortType=input  RightPortType=output  PseudoPeriodic=off  Frequencies=[]  Unit=m  AffineConversion=off
      settings: AttributesFormatString=UNITS=%<Unit>
  PS-Simulink Converter2 : nesl_utility/PS-Simulink Converter  PhysicalDomain=network_engine_domain  SubClassName=ps_output  LeftPortType=input  RightPortType=output  PseudoPeriodic=off  Frequencies=[]  Unit=m/s  AffineConversion=off
      settings: AttributesFormatString=UNITS=%<Unit>
  PS-Simulink Converter3 : nesl_utility/PS-Simulink Converter  PhysicalDomain=network_engine_domain  SubClassName=ps_output  LeftPortType=input  RightPortType=output  PseudoPeriodic=off  Frequencies=[]  Unit=m  AffineConversion=off
      settings: AttributesFormatString=UNITS=%<Unit>
  PS-Simulink Converter4 : nesl_utility/PS-Simulink Converter  PhysicalDomain=network_engine_domain  SubClassName=ps_output  LeftPortType=input  RightPortType=output  PseudoPeriodic=off  Frequencies=[]  Unit=m/s  AffineConversion=off
      settings: AttributesFormatString=UNITS=%<Unit>
  PS-Simulink Converter7 : nesl_utility/PS-Simulink Converter  PhysicalDomain=network_engine_domain  SubClassName=ps_output  LeftPortType=input  RightPortType=output  PseudoPeriodic=off  Frequencies=[]  Unit=rad  AffineConversion=off
      settings: AttributesFormatString=UNITS=%<Unit>
  PS-Simulink Converter8 : nesl_utility/PS-Simulink Converter  PhysicalDomain=network_engine_domain  SubClassName=ps_output  LeftPortType=input  RightPortType=output  PseudoPeriodic=off  Frequencies=[]  Unit=1  AffineConversion=off
      settings: AttributesFormatString=UNITS=%<Unit>
  Product1 : Product
  Radians to Degrees : simulink_extras/Transformations/Radians to Degrees
  Scope : Scope
  Selector1 : Selector  InputPortWidth=3  IndexOptions=Index vector (dialog)  Indices=3  OutputSizes=1
  Transform Sensor : sm_lib/Frames and Transforms/Transform Sensor  MeasurementFrame=World  SenseAngle=on  SenseAxis=on  SenseAngle1=off  SenseAngle2=off  SenseAngle3=off  SenseQ=off  SenseR=off  SenseOmegaX=off  SenseOmegaY=off  SenseOmegaZ=off  SenseOmega1=off  SenseOmega2=off  SenseOmega3=off  SenseQDot=off  SenseRDot=off  SenseAlphaX=off  SenseAlphaY=off  SenseAlphaZ=off  SenseAlpha1=off  SenseAlpha2=off  SenseAlpha3=off  SenseQDDot=off  SenseRDDot=off  SenseX=on  SenseY=on  SenseZ=off  SenseRad=off  SenseAzim=off  SenseDist=off  SenseInc=off  SenseXDot=on  SenseYDot=on  SenseZDot=off  SenseRadDot=off  SenseAzimDot=off  SenseDistDot=off  SenseIncDot=off  SenseXDDot=off  SenseYDDot=off  SenseZDDot=off  SenseRadDDot=off  SenseAzimDDot=off  SenseDistDDot=off  SenseIncDDot=off
  World Frame : sm_lib/Frames and Transforms/World Frame
  A : PMIOPort  Side=Left
  NA : Outport
  wires:
  PS-Simulink Converter2/1 -> Bus Creator/4  "vt_x"
  Bus Creator/1 -> NA/1
  PS-Simulink Converter1/1 -> Bus Creator/2  "pt_x"
  PS-Simulink Converter4/1 -> Bus Creator/5  "vt_y"
  PS-Simulink Converter3/1 -> Bus Creator/3  "pt_y"
  Radians to Degrees/1 -> Bus Creator/1, Scope/1  "ang_wrt_W"
  [TS_theta_RAD] -> Product1/1
  [TS_ax] -> Selector1/1
  Product1/1 -> [TS_SIGNED_theta_RAD]
  Selector1/1 -> Product1/2
  PS-Simulink Converter7/1 -> [TS_theta_RAD]  "ang_wrt_W"
  PS-Simulink Converter8/1 -> [TS_ax]  "TS_ax"
  [TS_SIGNED_theta_RAD] -> Radians to Degrees/1
  connections:
  A/RConn1 -- Transform Sensor/RConn1
  Transform Sensor/LConn1 -- World Frame/RConn1
  Transform Sensor/RConn7 -- PS-Simulink Converter4/LConn1
  PS-Simulink Converter2/LConn1 -- Transform Sensor/RConn6
  PS-Simulink Converter3/LConn1 -- Transform Sensor/RConn5
  PS-Simulink Converter1/LConn1 -- Transform Sensor/RConn4
  PS-Simulink Converter7/LConn1 -- Transform Sensor/RConn2
  PS-Simulink Converter8/LConn1 -- Transform Sensor/RConn3

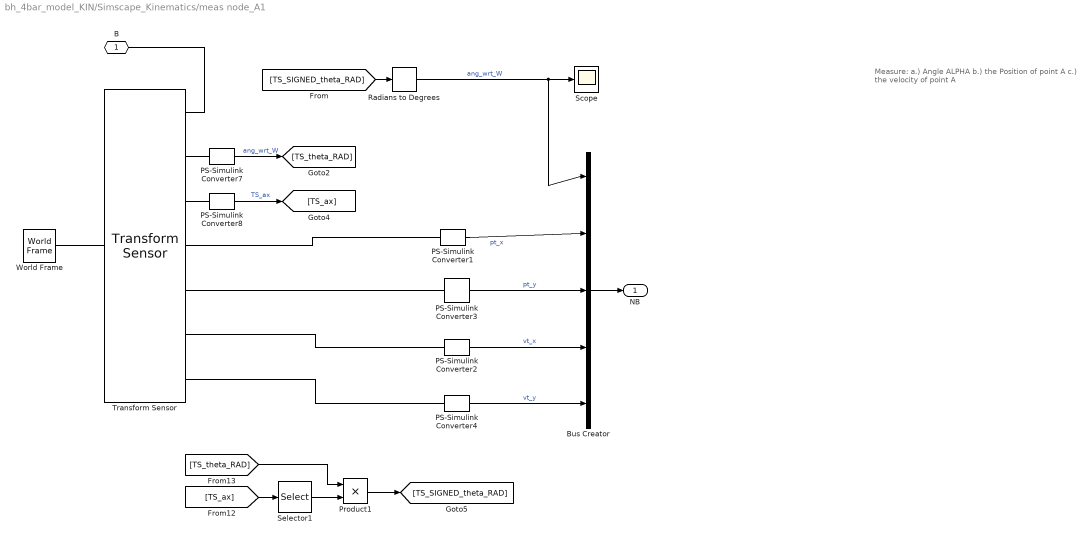
== system bh_4bar_model_KIN/Simscape_Kinematics/meas node_A1 ==
  note: Measure:
      | a.) Angle ALPHA
      | b.) the Position of point A
      | c.) the velocity of point A
  Bus Creator : BusCreator  Inputs=5
  PS-Simulink Converter1 : nesl_utility/PS-Simulink Converter  PhysicalDomain=network_engine_domain  SubClassName=ps_output  LeftPortType=input  RightPortType=output  PseudoPeriodic=off  Frequencies=[]  Unit=m  AffineConversion=off
      settings: AttributesFormatString=UNITS=%<Unit>
  PS-Simulink Converter2 : nesl_utility/PS-Simulink Converter  PhysicalDomain=network_engine_domain  SubClassName=ps_output  LeftPortType=input  RightPortType=output  PseudoPeriodic=off  Frequencies=[]  Unit=m/s  AffineConversion=off
      settings: AttributesFormatString=UNITS=%<Unit>
  PS-Simulink Converter3 : nesl_utility/PS-Simulink Converter  PhysicalDomain=network_engine_domain  SubClassName=ps_output  LeftPortType=input  RightPortType=output  PseudoPeriodic=off  Frequencies=[]  Unit=m  AffineConversion=off
      settings: AttributesFormatString=UNITS=%<Unit>
  PS-Simulink Converter4 : nesl_utility/PS-Simulink Converter  PhysicalDomain=network_engine_domain  SubClassName=ps_output  LeftPortType=input  RightPortType=output  PseudoPeriodic=off  Frequencies=[]  Unit=m/s  AffineConversion=off
      settings: AttributesFormatString=UNITS=%<Unit>
  PS-Simulink Converter7 : nesl_utility/PS-Simulink Converter  PhysicalDomain=network_engine_domain  SubClassName=ps_output  LeftPortType=input  RightPortType=output  PseudoPeriodic=off  Frequencies=[]  Unit=rad  AffineConversion=off
      settings: AttributesFormatString=UNITS=%<Unit>
  PS-Simulink Converter8 : nesl_utility/PS-Simulink Converter  PhysicalDomain=network_engine_domain  SubClassName=ps_output  LeftPortType=input  RightPortType=output  PseudoPeriodic=off  Frequencies=[]  Unit=1  AffineConversion=off
      settings: AttributesFormatString=UNITS=%<Unit>
  Product1 : Product
  Radians to Degrees : simulink_extras/Transformations/Radians to Degrees
  Scope : Scope
  Selector1 : Selector  InputPortWidth=3  IndexOptions=Index vector (dialog)  Indices=3  OutputSizes=1
  Transform Sensor : sm_lib/Frames and Transforms/Transform Sensor  MeasurementFrame=World  SenseAngle=on  SenseAxis=on  SenseAngle1=off  SenseAngle2=off  SenseAngle3=off  SenseQ=off  SenseR=off  SenseOmegaX=off  SenseOmegaY=off  SenseOmegaZ=off  SenseOmega1=off  SenseOmega2=off  SenseOmega3=off  SenseQDot=off  SenseRDot=off  SenseAlphaX=off  SenseAlphaY=off  SenseAlphaZ=off  SenseAlpha1=off  SenseAlpha2=off  SenseAlpha3=off  SenseQDDot=off  SenseRDDot=off  SenseX=on  SenseY=on  SenseZ=off  SenseRad=off  SenseAzim=off  SenseDist=off  SenseInc=off  SenseXDot=on  SenseYDot=on  SenseZDot=off  SenseRadDot=off  SenseAzimDot=off  SenseDistDot=off  SenseIncDot=off  SenseXDDot=off  SenseYDDot=off  SenseZDDot=off  SenseRadDDot=off  SenseAzimDDot=off  SenseDistDDot=off  SenseIncDDot=off
  World Frame : sm_lib/Frames and Transforms/World Frame
  B : PMIOPort  Side=Left
  NB : Outport
  wires:
  PS-Simulink Converter2/1 -> Bus Creator/4  "vt_x"
  Bus Creator/1 -> NB/1
  PS-Simulink Converter1/1 -> Bus Creator/2  "pt_x"
  PS-Simulink Converter4/1 -> Bus Creator/5  "vt_y"
  PS-Simulink Converter3/1 -> Bus Creator/3  "pt_y"
  Radians to Degrees/1 -> Bus Creator/1, Scope/1  "ang_wrt_W"
  [TS_theta_RAD] -> Product1/1
  [TS_ax] -> Selector1/1
  Product1/1 -> [TS_SIGNED_theta_RAD]
  Selector1/1 -> Product1/2
  PS-Simulink Converter7/1 -> [TS_theta_RAD]  "ang_wrt_W"
  PS-Simulink Converter8/1 -> [TS_ax]  "TS_ax"
  [TS_SIGNED_theta_RAD] -> Radians to Degrees/1
  connections:
  B/RConn1 -- Transform Sensor/RConn1
  Transform Sensor/LConn1 -- World Frame/RConn1
  Transform Sensor/RConn7 -- PS-Simulink Converter4/LConn1
  PS-Simulink Converter2/LConn1 -- Transform Sensor/RConn6
  PS-Simulink Converter3/LConn1 -- Transform Sensor/RConn5
  PS-Simulink Converter1/LConn1 -- Transform Sensor/RConn4
  PS-Simulink Converter7/LConn1 -- Transform Sensor/RConn2
  PS-Simulink Converter8/LConn1 -- Transform Sensor/RConn3

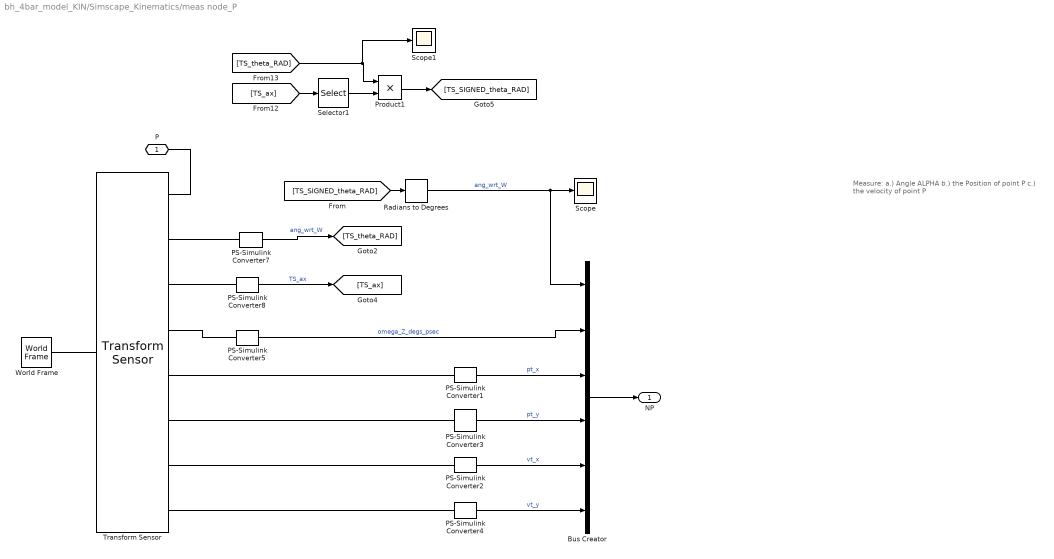
== system bh_4bar_model_KIN/Simscape_Kinematics/meas node_P ==
  note: Measure:
      | a.) Angle ALPHA
      | b.) the Position of point P
      | c.) the velocity of point P
  Bus Creator : BusCreator  Inputs=6
  PS-Simulink Converter1 : nesl_utility/PS-Simulink Converter  PhysicalDomain=network_engine_domain  SubClassName=ps_output  LeftPortType=input  RightPortType=output  PseudoPeriodic=off  Frequencies=[]  Unit=m  AffineConversion=off
      settings: AttributesFormatString=UNITS=%<Unit>
  PS-Simulink Converter2 : nesl_utility/PS-Simulink Converter  PhysicalDomain=network_engine_domain  SubClassName=ps_output  LeftPortType=input  RightPortType=output  PseudoPeriodic=off  Frequencies=[]  Unit=m/s  AffineConversion=off
      settings: AttributesFormatString=UNITS=%<Unit>
  PS-Simulink Converter3 : nesl_utility/PS-Simulink Converter  PhysicalDomain=network_engine_domain  SubClassName=ps_output  LeftPortType=input  RightPortType=output  PseudoPeriodic=off  Frequencies=[]  Unit=m  AffineConversion=off
      settings: AttributesFormatString=UNITS=%<Unit>
  PS-Simulink Converter4 : nesl_utility/PS-Simulink Converter  PhysicalDomain=network_engine_domain  SubClassName=ps_output  LeftPortType=input  RightPortType=output  PseudoPeriodic=off  Frequencies=[]  Unit=m/s  AffineConversion=off
      settings: AttributesFormatString=UNITS=%<Unit>
  PS-Simulink Converter5 : nesl_utility/PS-Simulink Converter  PhysicalDomain=network_engine_domain  SubClassName=ps_output  LeftPortType=input  RightPortType=output  PseudoPeriodic=off  Frequencies=[]  Unit=deg/s  AffineConversion=off
      settings: AttributesFormatString=UNITS=%<Unit>
  PS-Simulink Converter7 : nesl_utility/PS-Simulink Converter  PhysicalDomain=network_engine_domain  SubClassName=ps_output  LeftPortType=input  RightPortType=output  PseudoPeriodic=off  Frequencies=[]  Unit=rad  AffineConversion=off
      settings: AttributesFormatString=UNITS=%<Unit>
  PS-Simulink Converter8 : nesl_utility/PS-Simulink Converter  PhysicalDomain=network_engine_domain  SubClassName=ps_output  LeftPortType=input  RightPortType=output  PseudoPeriodic=off  Frequencies=[]  Unit=1  AffineConversion=off
      settings: AttributesFormatString=UNITS=%<Unit>
  Product1 : Product
  Radians to Degrees : simulink_extras/Transformations/Radians to Degrees
  Scope : Scope
  Scope1 : Scope
  Selector1 : Selector  InputPortWidth=3  IndexOptions=Index vector (dialog)  Indices=3  OutputSizes=1
  Transform Sensor : sm_lib/Frames and Transforms/Transform Sensor  MeasurementFrame=World  SenseAngle=on  SenseAxis=on  SenseAngle1=off  SenseAngle2=off  SenseAngle3=off  SenseQ=off  SenseR=off  SenseOmegaX=off  SenseOmegaY=off  SenseOmegaZ=on  SenseOmega1=off  SenseOmega2=off  SenseOmega3=off  SenseQDot=off  SenseRDot=off  SenseAlphaX=off  SenseAlphaY=off  SenseAlphaZ=off  SenseAlpha1=off  SenseAlpha2=off  SenseAlpha3=off  SenseQDDot=off  SenseRDDot=off  SenseX=on  SenseY=on  SenseZ=off  SenseRad=off  SenseAzim=off  SenseDist=off  SenseInc=off  SenseXDot=on  SenseYDot=on  SenseZDot=off  SenseRadDot=off  SenseAzimDot=off  SenseDistDot=off  SenseIncDot=off  SenseXDDot=off  SenseYDDot=off  SenseZDDot=off  SenseRadDDot=off  SenseAzimDDot=off  SenseDistDDot=off  SenseIncDDot=off
  World Frame : sm_lib/Frames and Transforms/World Frame
  P : PMIOPort  Side=Left
  NP : Outport
  wires:
  PS-Simulink Converter2/1 -> Bus Creator/5  "vt_x"
  Bus Creator/1 -> NP/1
  PS-Simulink Converter1/1 -> Bus Creator/3  "pt_x"
  PS-Simulink Converter4/1 -> Bus Creator/6  "vt_y"
  PS-Simulink Converter3/1 -> Bus Creator/4  "pt_y"
  Radians to Degrees/1 -> Bus Creator/1, Scope/1  "ang_wrt_W"
  [TS_theta_RAD] -> Scope1/1, Product1/1
  [TS_ax] -> Selector1/1
  Product1/1 -> [TS_SIGNED_theta_RAD]
  Selector1/1 -> Product1/2
  PS-Simulink Converter7/1 -> [TS_theta_RAD]  "ang_wrt_W"
  PS-Simulink Converter8/1 -> [TS_ax]  "TS_ax"
  [TS_SIGNED_theta_RAD] -> Radians to Degrees/1
  PS-Simulink Converter5/1 -> Bus Creator/2  "omega_Z_degs_psec"
  connections:
  Transform Sensor/RConn1 -- P/RConn1
  Transform Sensor/LConn1 -- World Frame/RConn1
  PS-Simulink Converter4/LConn1 -- Transform Sensor/RConn8
  PS-Simulink Converter2/LConn1 -- Transform Sensor/RConn7
  PS-Simulink Converter3/LConn1 -- Transform Sensor/RConn6
  PS-Simulink Converter1/LConn1 -- Transform Sensor/RConn5
  Transform Sensor/RConn2 -- PS-Simulink Converter7/LConn1
  PS-Simulink Converter8/LConn1 -- Transform Sensor/RConn3
  Transform Sensor/RConn4 -- PS-Simulink Converter5/LConn1

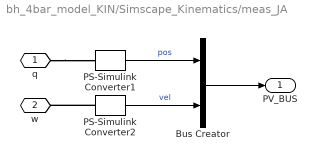
== system bh_4bar_model_KIN/Simscape_Kinematics/meas_JA ==
  Bus Creator : BusCreator  Inputs=2
  PS-Simulink Converter1 : nesl_utility/PS-Simulink Converter  PhysicalDomain=network_engine_domain  SubClassName=ps_output  LeftPortType=input  RightPortType=output  PseudoPeriodic=off  Frequencies=[]  Unit=deg  AffineConversion=off
  PS-Simulink Converter2 : nesl_utility/PS-Simulink Converter  PhysicalDomain=network_engine_domain  SubClassName=ps_output  LeftPortType=input  RightPortType=output  PseudoPeriodic=off  Frequencies=[]  Unit=deg/s  AffineConversion=off
  q : PMIOPort  Side=Left
  w : PMIOPort  Port=2  Side=Left
  PV_BUS : Outport
  wires:
  PS-Simulink Converter2/1 -> Bus Creator/2  "vel"
  PS-Simulink Converter1/1 -> Bus Creator/1  "pos"
  Bus Creator/1 -> PV_BUS/1
  connections:
  q/RConn1 -- PS-Simulink Converter1/LConn1
  PS-Simulink Converter2/LConn1 -- w/RConn1

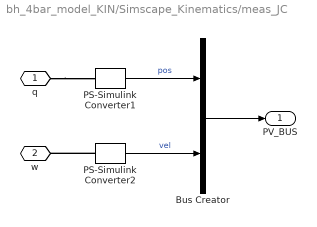
== system bh_4bar_model_KIN/Simscape_Kinematics/meas_JC ==
  Bus Creator : BusCreator  Inputs=2
  PS-Simulink Converter1 : nesl_utility/PS-Simulink Converter  PhysicalDomain=network_engine_domain  SubClassName=ps_output  LeftPortType=input  RightPortType=output  PseudoPeriodic=off  Frequencies=[]  Unit=deg  AffineConversion=off
      settings: AttributesFormatString=UNITS=%<Unit>
  PS-Simulink Converter2 : nesl_utility/PS-Simulink Converter  PhysicalDomain=network_engine_domain  SubClassName=ps_output  LeftPortType=input  RightPortType=output  PseudoPeriodic=off  Frequencies=[]  Unit=deg/s  AffineConversion=off
      settings: AttributesFormatString=UNITS=%<Unit>
  q : PMIOPort  Side=Left
  w : PMIOPort  Port=2  Side=Left
  PV_BUS : Outport
  wires:
  PS-Simulink Converter2/1 -> Bus Creator/2  "vel"
  PS-Simulink Converter1/1 -> Bus Creator/1  "pos"
  Bus Creator/1 -> PV_BUS/1
  connections:
  q/RConn1 -- PS-Simulink Converter1/LConn1
  PS-Simulink Converter2/LConn1 -- w/RConn1

== system bh_4bar_model_KIN/Simscape_Kinematics/meas_JD ==
  Bus Creator : BusCreator  Inputs=2
  PS-Simulink Converter1 : nesl_utility/PS-Simulink Converter  PhysicalDomain=network_engine_domain  SubClassName=ps_output  LeftPortType=input  RightPortType=output  PseudoPeriodic=off  Frequencies=[]  Unit=deg  AffineConversion=off
  PS-Simulink Converter2 : nesl_utility/PS-Simulink Converter  PhysicalDomain=network_engine_domain  SubClassName=ps_output  LeftPortType=input  RightPortType=output  PseudoPeriodic=off  Frequencies=[]  Unit=deg/s  AffineConversion=off
  q : PMIOPort  Side=Left
  w : PMIOPort  Port=2  Side=Left
  PV_BUS : Outport
  wires:
  PS-Simulink Converter2/1 -> Bus Creator/2  "vel"
  PS-Simulink Converter1/1 -> Bus Creator/1  "pos"
  Bus Creator/1 -> PV_BUS/1
  connections:
  q/RConn1 -- PS-Simulink Converter1/LConn1
  PS-Simulink Converter2/LConn1 -- w/RConn1
